simulink model "UAV_Gimbal_Stabilization_and_Moving_Target_Tracking"  (R2026a)
settings: Solver=VariableStepAuto  StopTime=100.0
libraries: slpidlib x2, simulink x2
settings Model: Creator=santiago  LastModifiedBy=santiago

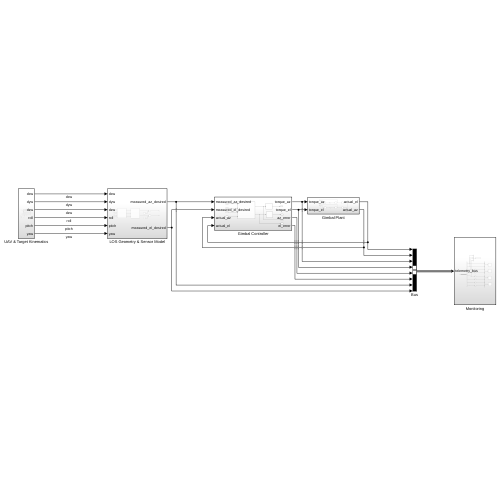
[thumbnail: Simulink's stored preview of the top-level diagram]
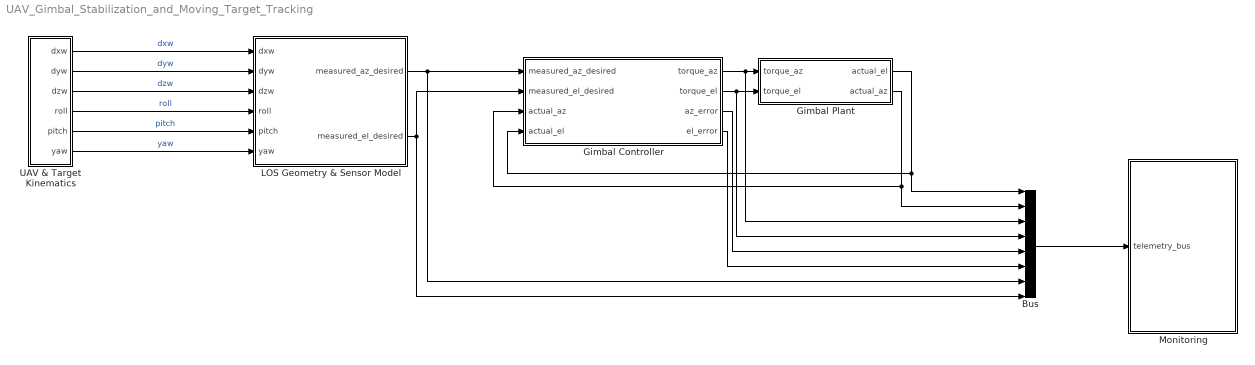
== system UAV_Gimbal_Stabilization_and_Moving_Target_Tracking ==
  Bus : BusCreator  Inputs=8
  Gimbal Controller : Subsystem
  Gimbal Plant : Subsystem
  LOS Geometry & Sensor Model : Subsystem
  Monitoring : Subsystem
  UAV & Target Kinematics : Subsystem
  wires:
  LOS Geometry & Sensor Model/1(measured_az_desired) -> Bus/7, Gimbal Controller/1(measured_az_desired)
  LOS Geometry & Sensor Model/2(measured_el_desired) -> Bus/8, Gimbal Controller/2(measured_el_desired)
  UAV & Target Kinematics/1(dxw) -> LOS Geometry & Sensor Model/1(dxw)  "dxw"
  UAV & Target Kinematics/2(dyw) -> LOS Geometry & Sensor Model/2(dyw)  "dyw"
  UAV & Target Kinematics/3(dzw) -> LOS Geometry & Sensor Model/3(dzw)  "dzw"
  UAV & Target Kinematics/4(roll) -> LOS Geometry & Sensor Model/4(roll)  "roll"
  UAV & Target Kinematics/5(pitch) -> LOS Geometry & Sensor Model/5(pitch)  "pitch"
  UAV & Target Kinematics/6(yaw) -> LOS Geometry & Sensor Model/6(yaw)  "yaw"
  Gimbal Controller/1(torque_az) -> Gimbal Plant/1(torque_az), Bus/3
  Gimbal Controller/2(torque_el) -> Bus/4, Gimbal Plant/2(torque_el)
  Gimbal Controller/3(az_error) -> Bus/5
  Gimbal Controller/4(el_error) -> Bus/6
  Bus/1 -> Monitoring/1(telemetry_bus)
  Gimbal Plant/2(actual_az) -> Bus/2, Gimbal Controller/3(actual_az)
  Gimbal Plant/1(actual_el) -> Bus/1, Gimbal Controller/4(actual_el)

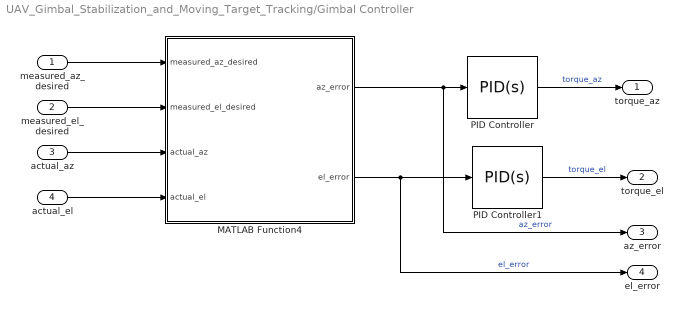
== system UAV_Gimbal_Stabilization_and_Moving_Target_Tracking/Gimbal Controller ==
  measured_az_desired : Inport
  measured_el_desired : Inport  Port=2
  actual_az : Inport  Port=3
  actual_el : Inport  Port=4
  MATLAB Function4 : MATLAB Function  TreatAsAtomicUnit=on
  PID Controller : slpidlib/PID Controller  Controller=PID  Form=Parallel  TimeDomain=Continuous-time  UseExternalTs=off  SampleTime=-1  IntegratorMethod=Forward Euler  FilterMethod=Forward Euler  ControllerParametersSource=internal  P=2  I=0.5  UseKiTs=off  D=0.20  UseExternalDerivativeSource=off  N=100  UseFilter=on  TunerSelectOption=Transfer Function Based (PID Tuner App)  InitialConditionSource=internal  InitialConditionForIntegrator=0  InitialConditionForFilter=0  DifferentiatorICPrevScaledInput=0  ExternalReset=none  TrackingMode=off  Kt=1  LimitOutput=on  SatLimitsSource=internal  UpperSaturationLimit=1.5  LowerSaturationLimit=-1.5  LinearizeAsGain=on  AntiWindupMode=back-calculation  Kb=1  LimitIntegrator=off  UpperIntegratorSaturationLimit=inf  LowerIntegratorSaturationLimit=-inf  POutMin=[]  POutMax=[]  IOutMin=[]  IOutMax=[]  DOutMin=[]  DOutMax=[]  NOutMin=[]  NOutMax=[]  SumOutMin=[]  SumOutMax=[]  SaturationOutMin=[]  SaturationOutMax=[]  PParamMin=[]  PParamMax=[]  IParamMin=[]  IParamMax=[]  DParamMin=[]  DParamMax=[]  NParamMin=[]  NParamMax=[]  KbParamMin=[]  KbParamMax=[]  KtParamMin=[]  KtParamMax=[]  KbOutMin=[]  KbOutMax=[]  KtOutMin=[]  KtOutMax=[]  IntegratorOutMin=[]  IntegratorOutMax=[]  FilterOutMin=[]  FilterOutMax=[]  SumI1OutMin=[]  SumI1OutMax=[]  SumI2OutMin=[]  SumI2OutMax=[]  SumI3OutMin=[]  SumI3OutMax=[]  SumI4OutMin=[]  SumI4OutMax=[]  SumDOutMin=[]  SumDOutMax=[]  DifferentiatorOutMin=[]  DifferentiatorOutMax=[]  FilterDiffOutCoefMin=[]  FilterDiffOutCoefMax=[]  ReciprocalOutMin=[]  ReciprocalOutMax=[]  SumDenOutMin=[]  SumDenOutMax=[]  SumNumOutMin=[]  SumNumOutMax=[]  DivideOutMin=[]  DivideOutMax=[]  UdiffTsProdOutMin=[]  UdiffTsProdOutMax=[]  NTsProdOutMin=[]  NTsProdOutMax=[]  UintegralTsProdOutMin=[]  UintegralTsProdOutMax=[]  UngainTsProdOutMin=[]  UngainTsProdOutMax=[]  ClampingZeroOutDataTypeStr=Inherit: Inherit via back propagation  ClampingZeroOutMin=[]  ClampingZeroOutMax=[]  FilterDenConstantOutDataTypeStr=Inherit: Inherit via back propagation  FilterDenConstantOutMin=[]  FilterDenConstantOutMax=[]  PCopyOutDataTypeStr=Inherit: Inherit via back propagation  PCopyOutMin=[]  PCopyOutMax=[]  NCopyOutDataTypeStr=Inherit: Inherit via back propagation  NCopyOutMin=[]  NCopyOutMax=[]  IntegratorContinuousStateAttributes=''  IntegratorStateMustResolveToSignalObject=off  IntegratorRTWStateStorageClass=Auto  FilterContinuousStateAttributes=''  FilterStateMustResolveToSignalObject=off  FilterRTWStateStorageClass=Auto  ParallelPVariant=InternalParameters  IdealPVariant=Disabled  IVariant=InternalParameters  DVariant=InternalParameters  IntegratorVariant=Continuous  SatVariant=Enabled  AWVariant=BackCalculation  PCopyVariant=Disabled  TRVariant=Disabled  FdbkBlocksVariant=Forward  IdealPFdbkVariant=Disabled  SatFdbkVariant=Disabled  DerivativeFilterVariant=ContFilter  NVariant=InternalParameters  NCopyVariant=Disabled  FilterICVariant=InternalICsFilter  IntegratorICVariant=InternalICs  ExternalResetVariant=Disabled  TRSumVariant=Passthrough  SumFdbkVariant=Disabled  SumVariant=Sum_PID  TsampFilterVariant=InternalTs  TsampNgainVariant=Passthrough  TsampIntegralVariant=Disabled_SignalSpec  ExternalSaturationOutDataTypeStr=Inherit: Same as second input  DerivativeSourceVariant=ErrorSignal  PreIntVariant=InternalPreInt
  PID Controller1 : slpidlib/PID Controller  Controller=PID  Form=Parallel  TimeDomain=Continuous-time  UseExternalTs=off  SampleTime=-1  IntegratorMethod=Forward Euler  FilterMethod=Forward Euler  ControllerParametersSource=internal  P=1.8  I=0.4  UseKiTs=off  D=0.18  UseExternalDerivativeSource=off  N=100  UseFilter=on  TunerSelectOption=Transfer Function Based (PID Tuner App)  InitialConditionSource=internal  InitialConditionForIntegrator=0  InitialConditionForFilter=0  DifferentiatorICPrevScaledInput=0  ExternalReset=none  TrackingMode=off  Kt=1  LimitOutput=on  SatLimitsSource=internal  UpperSaturationLimit=1.5  LowerSaturationLimit=-1.5  LinearizeAsGain=on  AntiWindupMode=back-calculation  Kb=1  LimitIntegrator=off  UpperIntegratorSaturationLimit=inf  LowerIntegratorSaturationLimit=-inf  POutMin=[]  POutMax=[]  IOutMin=[]  IOutMax=[]  DOutMin=[]  DOutMax=[]  NOutMin=[]  NOutMax=[]  SumOutMin=[]  SumOutMax=[]  SaturationOutMin=[]  SaturationOutMax=[]  PParamMin=[]  PParamMax=[]  IParamMin=[]  IParamMax=[]  DParamMin=[]  DParamMax=[]  NParamMin=[]  NParamMax=[]  KbParamMin=[]  KbParamMax=[]  KtParamMin=[]  KtParamMax=[]  KbOutMin=[]  KbOutMax=[]  KtOutMin=[]  KtOutMax=[]  IntegratorOutMin=[]  IntegratorOutMax=[]  FilterOutMin=[]  FilterOutMax=[]  SumI1OutMin=[]  SumI1OutMax=[]  SumI2OutMin=[]  SumI2OutMax=[]  SumI3OutMin=[]  SumI3OutMax=[]  SumI4OutMin=[]  SumI4OutMax=[]  SumDOutMin=[]  SumDOutMax=[]  DifferentiatorOutMin=[]  DifferentiatorOutMax=[]  FilterDiffOutCoefMin=[]  FilterDiffOutCoefMax=[]  ReciprocalOutMin=[]  ReciprocalOutMax=[]  SumDenOutMin=[]  SumDenOutMax=[]  SumNumOutMin=[]  SumNumOutMax=[]  DivideOutMin=[]  DivideOutMax=[]  UdiffTsProdOutMin=[]  UdiffTsProdOutMax=[]  NTsProdOutMin=[]  NTsProdOutMax=[]  UintegralTsProdOutMin=[]  UintegralTsProdOutMax=[]  UngainTsProdOutMin=[]  UngainTsProdOutMax=[]  ClampingZeroOutDataTypeStr=Inherit: Inherit via back propagation  ClampingZeroOutMin=[]  ClampingZeroOutMax=[]  FilterDenConstantOutDataTypeStr=Inherit: Inherit via back propagation  FilterDenConstantOutMin=[]  FilterDenConstantOutMax=[]  PCopyOutDataTypeStr=Inherit: Inherit via back propagation  PCopyOutMin=[]  PCopyOutMax=[]  NCopyOutDataTypeStr=Inherit: Inherit via back propagation  NCopyOutMin=[]  NCopyOutMax=[]  IntegratorContinuousStateAttributes=''  IntegratorStateMustResolveToSignalObject=off  IntegratorRTWStateStorageClass=Auto  FilterContinuousStateAttributes=''  FilterStateMustResolveToSignalObject=off  FilterRTWStateStorageClass=Auto  ParallelPVariant=InternalParameters  IdealPVariant=Disabled  IVariant=InternalParameters  DVariant=InternalParameters  IntegratorVariant=Continuous  SatVariant=Enabled  AWVariant=BackCalculation  PCopyVariant=Disabled  TRVariant=Disabled  FdbkBlocksVariant=Forward  IdealPFdbkVariant=Disabled  SatFdbkVariant=Disabled  DerivativeFilterVariant=ContFilter  NVariant=InternalParameters  NCopyVariant=Disabled  FilterICVariant=InternalICsFilter  IntegratorICVariant=InternalICs  ExternalResetVariant=Disabled  TRSumVariant=Passthrough  SumFdbkVariant=Disabled  SumVariant=Sum_PID  TsampFilterVariant=InternalTs  TsampNgainVariant=Passthrough  TsampIntegralVariant=Disabled_SignalSpec  ExternalSaturationOutDataTypeStr=Inherit: Same as second input  DerivativeSourceVariant=ErrorSignal  PreIntVariant=InternalPreInt
  torque_az : Outport
  torque_el : Outport  Port=2
  az_error : Outport  Port=3
  el_error : Outport  Port=4
  wires:
  PID Controller/1 -> torque_az/1  "torque_az"
  measured_az_desired/1 -> MATLAB Function4/1(measured_az_desired)
  actual_az/1 -> MATLAB Function4/3(actual_az)
  actual_el/1 -> MATLAB Function4/4(actual_el)
  PID Controller1/1 -> torque_el/1  "torque_el"
  measured_el_desired/1 -> MATLAB Function4/2(measured_el_desired)
  MATLAB Function4/1(az_error) -> az_error/1, PID Controller/1  "az_error"
  MATLAB Function4/2(el_error) -> el_error/1, PID Controller1/1  "el_error"

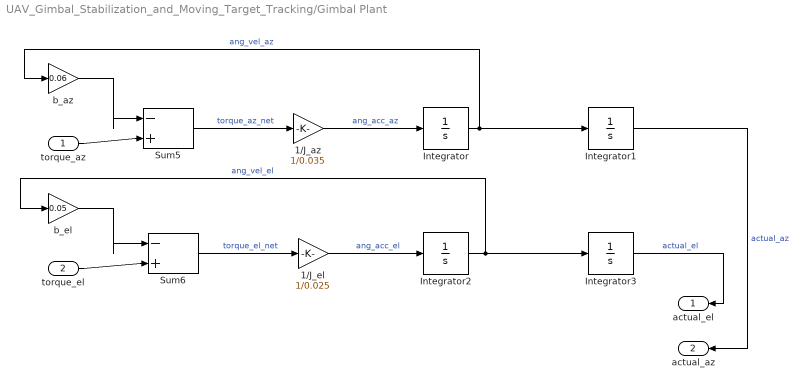
== system UAV_Gimbal_Stabilization_and_Moving_Target_Tracking/Gimbal Plant ==
  torque_az : Inport
  torque_el : Inport  Port=2
  1/J_az : Gain  Gain=1/0.035
  1/J_el : Gain  Gain=1/0.025
  Integrator : Integrator  LimitOutput=on  UpperSaturationLimit=deg2rad(120)  LowerSaturationLimit=-deg2rad(120)
  Integrator1 : Integrator  UpperSaturationLimit=deg2rad(160)  LowerSaturationLimit=-deg2rad(160)
  Integrator2 : Integrator  LimitOutput=on  UpperSaturationLimit=deg2rad(120)  LowerSaturationLimit=-deg2rad(120)
  Integrator3 : Integrator  LimitOutput=on  UpperSaturationLimit=deg2rad(30)  LowerSaturationLimit=-deg2rad(90)
  Sum5 : Sum  Inputs=|-+
  Sum6 : Sum  Inputs=|-+
  b_az : Gain  Gain=0.06
  b_el : Gain  Gain=0.05
  actual_el : Outport
  actual_az : Outport  Port=2
  wires:
  b_az/1 -> Sum5/1
  1/J_az/1 -> Integrator/1  "ang_acc_az"
  Integrator/1 -> b_az/1, Integrator1/1  "ang_vel_az"
  Sum5/1 -> 1/J_az/1  "torque_az_net"
  1/J_el/1 -> Integrator2/1  "ang_acc_el"
  Integrator2/1 -> b_el/1, Integrator3/1  "ang_vel_el"
  torque_az/1 -> Sum5/2
  Integrator1/1 -> actual_az/1  "actual_az"
  b_el/1 -> Sum6/1
  Integrator3/1 -> actual_el/1  "actual_el"
  Sum6/1 -> 1/J_el/1  "torque_el_net"
  torque_el/1 -> Sum6/2

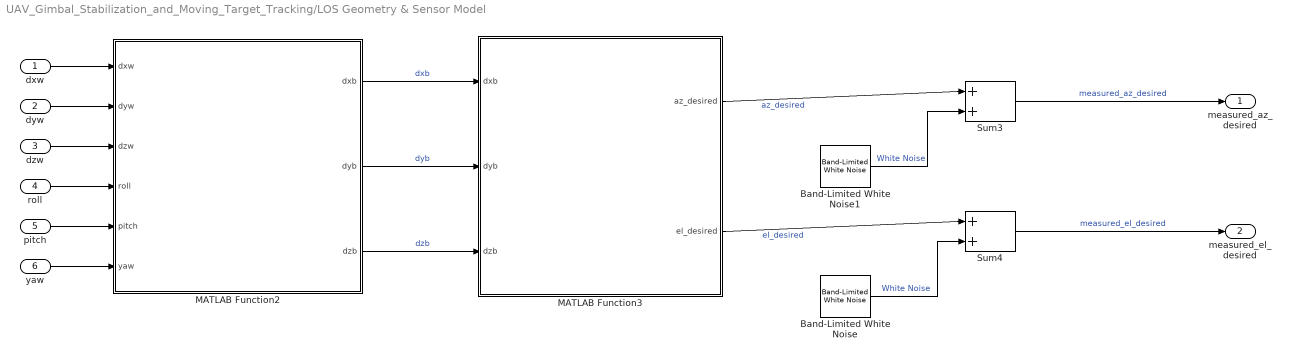
== system UAV_Gimbal_Stabilization_and_Moving_Target_Tracking/LOS Geometry & Sensor Model ==
  dxw : Inport
  dyw : Inport  Port=2
  dzw : Inport  Port=3
  roll : Inport  Port=4
  pitch : Inport  Port=5
  yaw : Inport  Port=6
  Band-Limited White Noise : simulink/Sources/Band-Limited White Noise  Cov=[(0.05*pi/180)^2 * 0.01]  Ts=0.01  seed=[23341]
  Band-Limited White Noise1 : simulink/Sources/Band-Limited White Noise  Cov=[(0.05*pi/180)^2 * 0.01]  Ts=0.01  seed=[23341]
  MATLAB Function2 : MATLAB Function  TreatAsAtomicUnit=on
  MATLAB Function3 : MATLAB Function  TreatAsAtomicUnit=on
  Sum3 : Sum  Inputs=|++
  Sum4 : Sum  Inputs=|++
  measured_az_desired : Outport
  measured_el_desired : Outport  Port=2
  wires:
  yaw/1 -> MATLAB Function2/6(yaw)
  dzw/1 -> MATLAB Function2/3(dzw)
  MATLAB Function2/3(dzb) -> MATLAB Function3/3(dzb)  "dzb"
  MATLAB Function3/1(az_desired) -> Sum3/1  "az_desired"
  Sum4/1 -> measured_el_desired/1  "measured_el_desired"
  dyw/1 -> MATLAB Function2/2(dyw)
  MATLAB Function2/1(dxb) -> MATLAB Function3/1(dxb)  "dxb"
  pitch/1 -> MATLAB Function2/5(pitch)
  MATLAB Function3/2(el_desired) -> Sum4/1  "el_desired"
  roll/1 -> MATLAB Function2/4(roll)
  Sum3/1 -> measured_az_desired/1  "measured_az_desired"
  Band-Limited White Noise/1 -> Sum4/2  "White Noise"
  MATLAB Function2/2(dyb) -> MATLAB Function3/2(dyb)  "dyb"
  Band-Limited White Noise1/1 -> Sum3/2  "White Noise"
  dxw/1 -> MATLAB Function2/1(dxw)

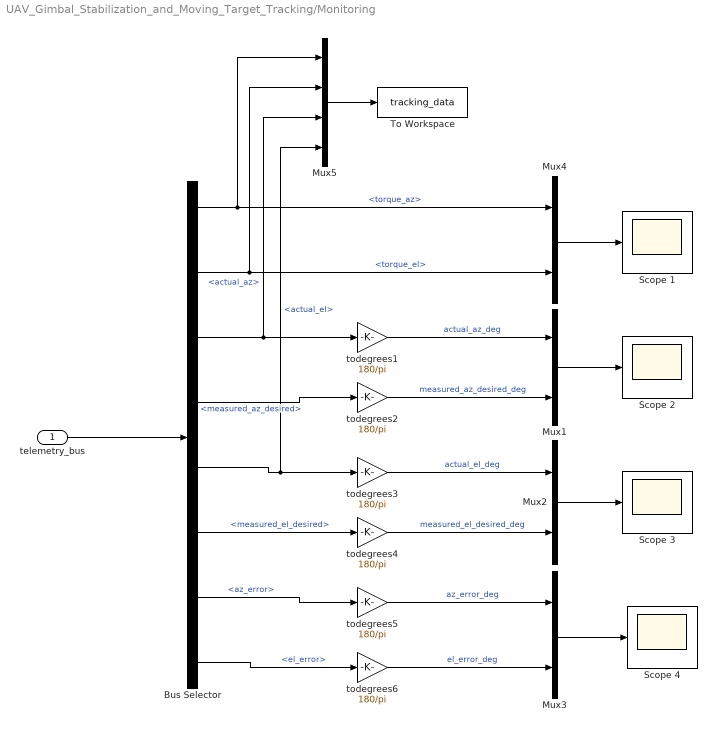
== system UAV_Gimbal_Stabilization_and_Moving_Target_Tracking/Monitoring ==
  telemetry_bus : Inport
  Bus Selector : BusSelector  OutputSignals=torque_az,torque_el,actual_az,measured_az_desired,actual_el,measured_el_desired,az_error,el_error
  Mux{1..4} (4 alike) : Mux  Inputs=2
  Mux5 : Mux
  Scope {1..4} (4 alike) : Scope
      Scope 1 settings: ActiveDisplayYMinimum=-2.4555166104171589  ActiveDisplayYMaximum=2.8211099745437807  DataLoggingVariableName=ScopeData3
      Scope 2 settings: ActiveDisplayYMinimum=-110.13109647701603  ActiveDisplayYMaximum=141.06451187801019
      Scope 3 settings: ActiveDisplayYMinimum=-107.25764906935508  ActiveDisplayYMaximum=26.624097853225472
      Scope 4 settings: ActiveDisplayYMinimum=-52.458731607953737  ActiveDisplayYMaximum=28.261247933013479  DataLoggingVariableName=ScopeData2
  To Workspace : ToWorkspace  VariableName=tracking_data  SaveFormat=Timeseries  SampleTime=-1
  todegrees{1..6} (6 alike) : Gain  Gain=180/pi
  wires:
  todegrees5/1 -> Mux3/1  "az_error_deg"
  todegrees6/1 -> Mux3/2  "el_error_deg"
  todegrees4/1 -> Mux2/2  "measured_el_desired_deg"
  todegrees1/1 -> Mux1/1  "actual_az_deg"
  Mux2/1 -> Scope 3/1
  Mux3/1 -> Scope 4/1
  todegrees2/1 -> Mux1/2  "measured_az_desired_deg"
  todegrees3/1 -> Mux2/1  "actual_el_deg"
  Mux1/1 -> Scope 2/1
  Mux4/1 -> Scope 1/1
  telemetry_bus/1 -> Bus Selector/1
  Bus Selector/4 -> todegrees2/1  "<measured_az_desired>"
  Bus Selector/7 -> todegrees5/1  "<az_error>"
  Bus Selector/6 -> todegrees4/1  "<measured_el_desired>"
  Bus Selector/5 -> Mux5/4, todegrees3/1  "<actual_el>"
  Bus Selector/8 -> todegrees6/1  "<el_error>"
  Bus Selector/2 -> Mux5/2, Mux4/2  "<torque_el>"
  Bus Selector/3 -> Mux5/3, todegrees1/1  "<actual_az>"
  Bus Selector/1 -> Mux5/1, Mux4/1  "<torque_az>"
  Mux5/1 -> To Workspace/1

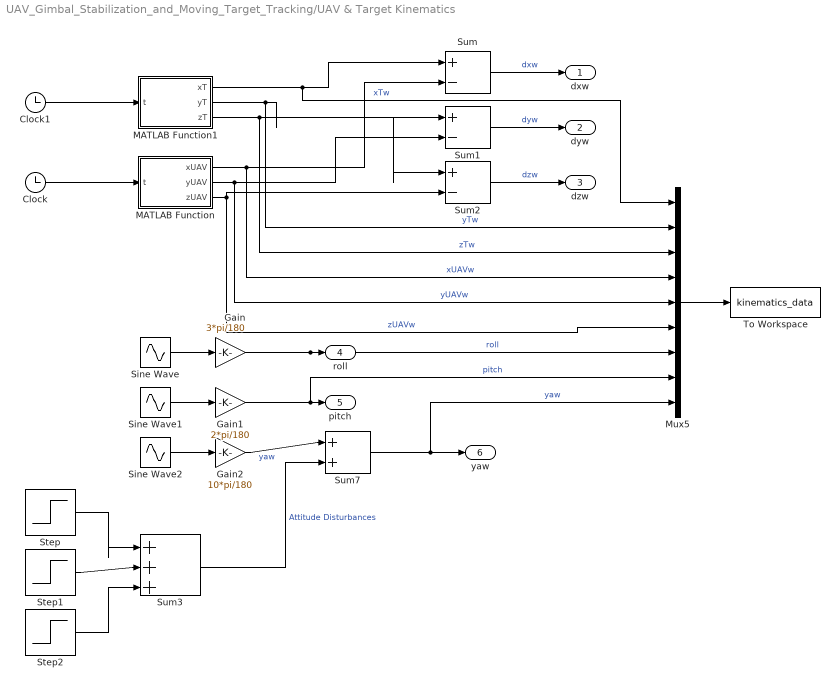
== system UAV_Gimbal_Stabilization_and_Moving_Target_Tracking/UAV & Target Kinematics ==
  Clock : Clock
  Clock1 : Clock
  Gain : Gain  Gain=3*pi/180
  Gain1 : Gain  Gain=2*pi/180
  Gain2 : Gain  Gain=10*pi/180
  MATLAB Function : MATLAB Function  TreatAsAtomicUnit=on
  MATLAB Function1 : MATLAB Function  TreatAsAtomicUnit=on
  Mux5 : Mux  Inputs=9
  Sine Wave : Sin  Frequency=1.4  SampleTime=0
  Sine Wave1 : Sin  Frequency=0.8  SampleTime=0
  Sine Wave2 : Sin  Frequency=0.05  SampleTime=0
  Step : Step  Time=30  FinalValue=deg2rad(12)  SampleTime=0
  Step1 : Step  Time=60  FinalValue=deg2rad(-10)  SampleTime=0
  Step2 : Step  Time=70  FinalValue=deg2rad(5)  SampleTime=0
  Sum : Sum  Inputs=|+-
  Sum1 : Sum  Inputs=|+-
  Sum2 : Sum  Inputs=|+-
  Sum3 : Sum  Inputs=|+++
  Sum7 : Sum  Inputs=|++
  To Workspace : ToWorkspace  VariableName=kinematics_data  SaveFormat=Timeseries  SampleTime=-1
  dxw : Outport
  dyw : Outport  Port=2
  dzw : Outport  Port=3
  roll : Outport  Port=4
  pitch : Outport  Port=5
  yaw : Outport  Port=6
  wires:
  Sum7/1 -> Mux5/9, yaw/1  "yaw"
  Sine Wave2/1 -> Gain2/1
  Sum2/1 -> dzw/1  "dzw"
  Gain1/1 -> Mux5/8, pitch/1  "pitch"
  Sum1/1 -> dyw/1  "dyw"
  Sum/1 -> dxw/1  "dxw"
  MATLAB Function1/1(xT) -> Mux5/1, Sum/1  "xTw"
  Gain/1 -> Mux5/7, roll/1  "roll"
  Clock/1 -> MATLAB Function/1(t)
  MATLAB Function1/3(zT) -> Mux5/3, Sum2/1  "zTw"
  MATLAB Function/1(xUAV) -> Mux5/4, Sum/2  "xUAVw"
  MATLAB Function/2(yUAV) -> Mux5/5, Sum1/2  "yUAVw"
  MATLAB Function/3(zUAV) -> Mux5/6, Sum2/2  "zUAVw"
  MATLAB Function1/2(yT) -> Mux5/2, Sum1/1  "yTw"
  Clock1/1 -> MATLAB Function1/1(t)
  Sine Wave/1 -> Gain/1
  Sine Wave1/1 -> Gain1/1
  Mux5/1 -> To Workspace/1
  Gain2/1 -> Sum7/1  "yaw"
  Step1/1 -> Sum3/2
  Step/1 -> Sum3/1
  Step2/1 -> Sum3/3
  Sum3/1 -> Sum7/2  "Attitude Disturbances"

== matlab function UAV_Gimbal_Stabilization_and_Moving_Target_Tracking/UAV & Target Kinematics/MATLAB Function1 ==
  data: t input; xT output; yT output; zT output
function [xT, yT, zT] = target_motion(t)

xT = 400 + 15*t;
yT = 200 + 300*sin(0.09*t);
zT = 0;

end

== matlab function UAV_Gimbal_Stabilization_and_Moving_Target_Tracking/UAV & Target Kinematics/MATLAB Function ==
  data: t input; xUAV output; yUAV output; zUAV output
function [xUAV, yUAV, zUAV] = UAV_trajectory(t)

xUAV = 20*t;
yUAV = 200*sin(0.03*t);
zUAV = 500 + 70*sin(0.1*t);

end

== matlab function UAV_Gimbal_Stabilization_and_Moving_Target_Tracking/LOS Geometry & Sensor Model/MATLAB Function2 ==
  data: dxb output; dxw input; dyb output; dzb output; dyw input; dzw input; roll input; pitch input; yaw input
function [dxb, dyb, dzb] = world_to_body_transformation(dxw, dyw, dzw, roll, pitch, yaw)

% Rotation around x-axis (roll)
Rx = [1,       0,          0;
    0, cos(roll), -sin(roll);
    0, sin(roll),  cos(roll)];

% Rotation around y-axis (pitch)
Ry = [ cos(pitch), 0, sin(pitch);
    0,          1, 0;
    -sin(pitch), 0, cos(pitch)];

% Rotation around z-axis (yaw)
Rz = [cos(yaw), -sin(yaw), 0;
    sin(yaw),  cos(yaw), 0;
    0,         0,        1];

% Body -> World rotation matrix
R = Rz * Ry * Rx;

% Relative target vector in world coordinates
rW = [dxw;
    dyw;
    dzw];

% World -> Body transformation
rB = R' * rW;

% Individual outputs
dxb = rB(1);
dyb = rB(2);
dzb = rB(3);

end

== matlab function UAV_Gimbal_Stabilization_and_Moving_Target_Tracking/LOS Geometry & Sensor Model/MATLAB Function3 ==
  data: dxb input; az_desired output; el_desired output; dyb input; dzb input
function [az_desired, el_desired] = LOS_geometry(dxb, dyb, dzb)

% Desired azimuth angle
az_desired = atan2(dyb, dxb);

% Horizontal distance between UAV and target
r_horizontal = sqrt(dxb^2 + dyb^2);

% Desired elevation angle
el_desired = atan2(dzb, r_horizontal);

end

== matlab function UAV_Gimbal_Stabilization_and_Moving_Target_Tracking/Gimbal Controller/MATLAB Function4 ==
  data: measured_az_desired input; az_error output; el_error output; measured_el_desired input; actual_az input; actual_el input
function [az_error, el_error] = angular_error(measured_az_desired, measured_el_desired, actual_az, actual_el)

% Angular error in azimuth
az_error = atan2(sin(measured_az_desired - actual_az), cos(measured_az_desired - actual_az));

% Angular error in elevation
el_error = measured_el_desired - actual_el;

end
